simulink model "compressionGainBlock"  (R2019a)
settings: Solver=VariableStepAuto  StartTime=0.0  StopTime=t_end  RelTol=1e-3
InitFcn:
  | clear;
  | [sig, fs] = audioread('UnitStepVolumeTest.wav');
  | [Gain_Table, xp_spacing, max_gain] = ...
  |    Compression_Wrapper(fs, 0, 1, [1], [10], 85, 1);
  | Ts = 1/fs;
  | tt = (0:length(sig)-1)./fs;
  | t_end = tt(end);
  | sig_in = [tt', sig.*max_gain];
  | 
  | Table_Fill = zeros(1,length(tt))';
  | Table_Fill(1:64) = Gain_Table;
  | Table_Fill = [tt', Table_Fill];
  | Fill_Valid = zeros(1,length(tt))';
  | Fill_Valid(1:64) = ones(1,64)';
  | Fill_Valid = boolean(Fill_Valid);
  | Fill_Valid = [tt', Fill_Valid];
  | 
  | Reset = [tt', boolean(zeros(1,length(tt)))'];
  | 
  | t_att = 0.2; s_att = t_att*fs;
  | t_rel = 2.0; s_rel = t_rel*fs;
  | r_att = nthroot(0.1, s_att);
  | r_rel = nthroot(0.1, s_rel);
values from neighbouring files (symbols this model uses):
  sig = sig * 10.^(.05*adjustdB)    [loadwavfile.m]    (also in testing.m = X_sweep(Volume,:)')
  xp_spacing = (X_high-X_thresh)*max_gain_prescript/63    [Compression_Wrapper.m]
libraries: hdlsllib x2, simulink x1
settings Model: Creator=Bailey  LastModifiedBy=Bailey

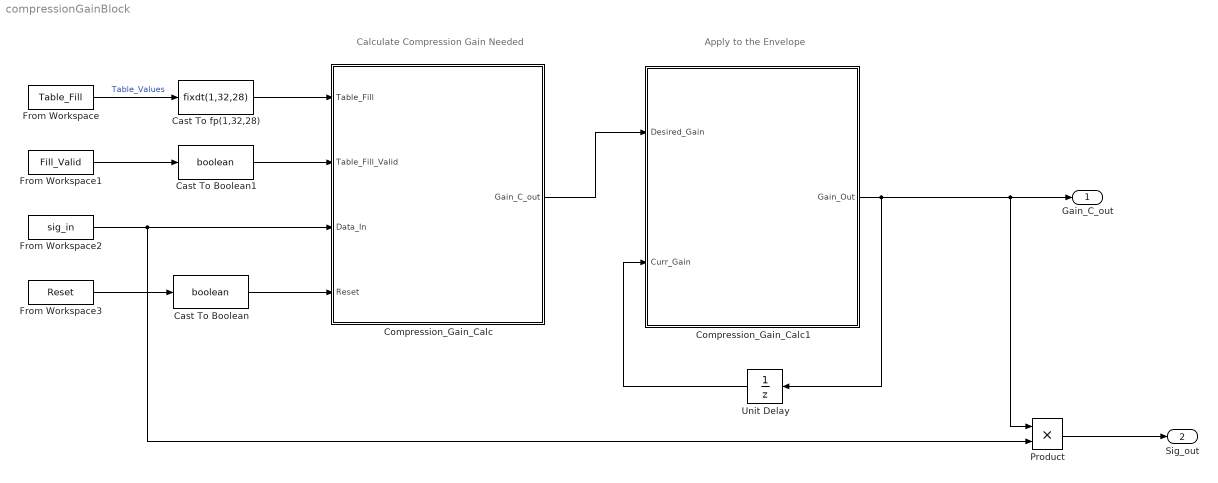
== system compressionGainBlock ==
  note: Apply to the Envelope
  note: Calculate Compression Gain Needed
  Cast To Boolean : DataTypeConversion  OutDataTypeStr=boolean
  Cast To Boolean1 : DataTypeConversion  OutDataTypeStr=boolean
  Cast To fp(1,32,28) : DataTypeConversion  OutDataTypeStr=fixdt(1,32,28)
  Compression_Gain_Calc : Subsystem
  Compression_Gain_Calc1 : Subsystem
  From Workspace : FromWorkspace  VariableName=Table_Fill  SampleTime=Ts  Interpolate=off  OutputAfterFinalValue=Setting to zero
  From Workspace1 : FromWorkspace  VariableName=Fill_Valid  SampleTime=Ts  OutputAfterFinalValue=Setting to zero
  From Workspace2 : FromWorkspace  VariableName=sig_in  SampleTime=Ts  Interpolate=off  OutputAfterFinalValue=Setting to zero
  From Workspace3 : FromWorkspace  VariableName=Reset  SampleTime=Ts  Interpolate=off  OutputAfterFinalValue=Setting to zero
  Product : Product
  Unit Delay : UnitDelay  InitialCondition=1  SampleTime=-1  HasFrameUpgradeWarning=on
  Gain_C_out : Outport
  Sig_out : Outport  Port=2
  wires:
  From Workspace2/1 -> Product/2, Compression_Gain_Calc/3(Data_In)
  From Workspace3/1 -> Cast To Boolean/1
  Cast To Boolean/1 -> Compression_Gain_Calc/4(Reset)
  From Workspace1/1 -> Cast To Boolean1/1
  Cast To Boolean1/1 -> Compression_Gain_Calc/2(Table_Fill_Valid)
  Cast To fp(1,32,28)/1 -> Compression_Gain_Calc/1(Table_Fill)
  From Workspace/1 -> Cast To fp(1,32,28)/1  "Table_Values"
  Compression_Gain_Calc/1(Gain_C_out) -> Compression_Gain_Calc1/1(Desired_Gain)
  Compression_Gain_Calc1/1(Gain_Out) -> Product/1, Gain_C_out/1, Unit Delay/1
  Unit Delay/1 -> Compression_Gain_Calc1/2(Curr_Gain)
  Product/1 -> Sig_out/1

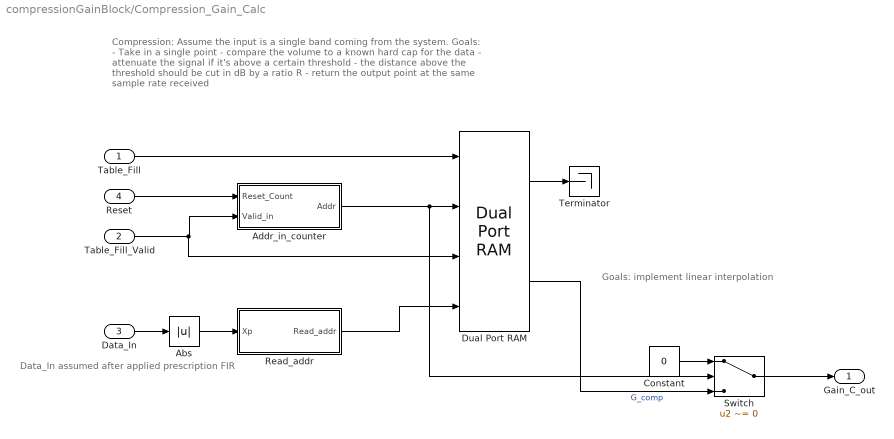
== system compressionGainBlock/Compression_Gain_Calc ==
  note: Goals: implement linear interpolation
  note: Data_In assumed after applied prescription FIR
  note: Compression: Assume the input is a single band coming from the system.
      |
      | Goals:
      | 	- Take in a single point
      | 	- compare the volume to a known hard cap for the data
      | 	- attenuate the signal if it's above a certain threshold
      | 		- the distance above the threshold should be cut in dB by a ratio R
      | 	- return the output point at the same sample rate received
  Table_Fill : Inport
  Table_Fill_Valid : Inport  Port=2
  Data_In : Inport  Port=3
  Reset : Inport  Port=4
  Abs : Abs
  Addr_in_counter : Subsystem
  Constant : Constant  Value=0  SampleTime=-1
  Dual Port RAM : hdlsllib/HDL RAMs/Dual Port RAM  ram_size=6
      settings: SourceProductName=Simulink  SourceProductBaseCode=SL
  Read_addr : Subsystem
  Switch : Switch  Criteria=u2 ~= 0  Threshold=63  ZeroCross=off
  Terminator : Terminator
  Gain_C_out : Outport
  wires:
  Reset/1 -> Addr_in_counter/1(Reset_Count)
  Dual Port RAM/1 -> Terminator/1
  Constant/1 -> Switch/1
  Switch/1 -> Gain_C_out/1
  Table_Fill/1 -> Dual Port RAM/1
  Table_Fill_Valid/1 -> Dual Port RAM/3, Addr_in_counter/2(Valid_in)
  Addr_in_counter/1(Addr) -> Switch/2, Dual Port RAM/2
  Dual Port RAM/2 -> Switch/3  "G_comp"
  Read_addr/1(Read_addr) -> Dual Port RAM/4
  Abs/1 -> Read_addr/1(Xp)
  Data_In/1 -> Abs/1

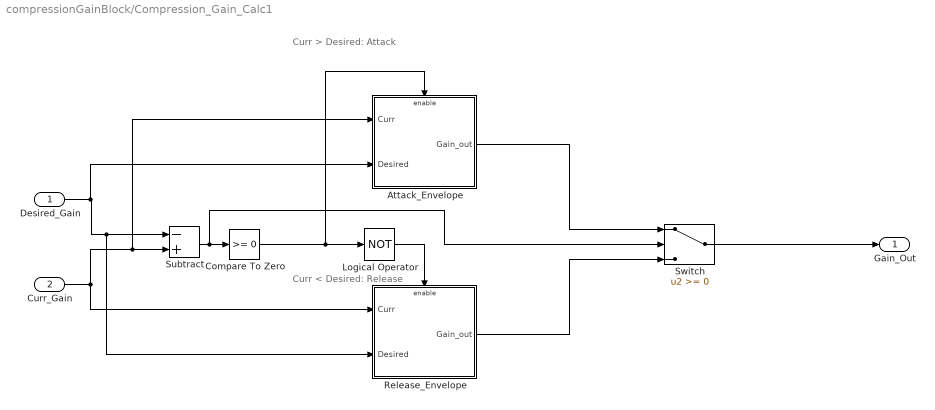
== system compressionGainBlock/Compression_Gain_Calc1 ==
  note: Curr > Desired:
      | Attack
  note: Curr < Desired:
      | Release
  Desired_Gain : Inport
  Curr_Gain : Inport  Port=2
  Attack_Envelope : Subsystem  TreatAsAtomicUnit=on
  Compare To Zero : simulink/Logic and Bit Operations/Compare To Zero  relop=>=  OutDataTypeStr=boolean
  Logical Operator : Logic  Operator=NOT  AllPortsSameDT=off  OutDataTypeStr=boolean
  Release_Envelope : Subsystem  TreatAsAtomicUnit=on
  Subtract : Sum  Inputs=-+
  Switch : Switch
  Gain_Out : Outport
  wires:
  Desired_Gain/1 -> Attack_Envelope/2(Desired), Release_Envelope/2(Desired), Subtract/1
  Curr_Gain/1 -> Attack_Envelope/1(Curr), Subtract/2, Release_Envelope/1(Curr)
  Subtract/1 -> Switch/2, Compare To Zero/1
  Compare To Zero/1 -> Attack_Envelope/Enable, Logical Operator/1
  Logical Operator/1 -> Release_Envelope/Enable
  Switch/1 -> Gain_Out/1
  Attack_Envelope/1(Gain_out) -> Switch/1
  Release_Envelope/1(Gain_out) -> Switch/3

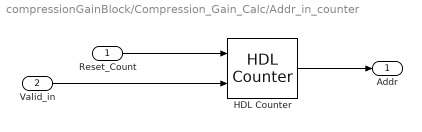
== system compressionGainBlock/Compression_Gain_Calc/Addr_in_counter ==
  Reset_Count : Inport
  Valid_in : Inport  Port=2
  HDL Counter : hdlsllib/Sources/HDL Counter  CountType=Count limited  CountInit=0  CountStep=1  CountMax=63  CountFromType=Initial value  CountFrom=0  CountResetPort=on  CountLoadPort=off  CountEnbPort=on  CountDirPort=off  CountDataType=Unsigned  CountWordLen=6  CountFracLen=0  CountSampTime=1
      settings: SourceProductName=Simulink
  Addr : Outport
  wires:
  Valid_in/1 -> HDL Counter/2
  Reset_Count/1 -> HDL Counter/1
  HDL Counter/1 -> Addr/1

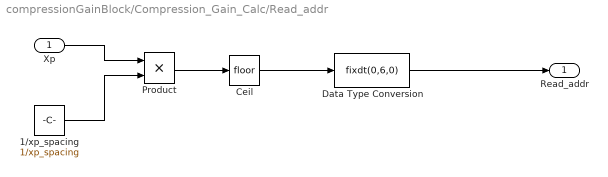
== system compressionGainBlock/Compression_Gain_Calc/Read_addr ==
  Xp : Inport
  1/xp_spacing : Constant  Value=1/xp_spacing  SampleTime=-1
  Ceil : Rounding
  Data Type Conversion : DataTypeConversion  OutDataTypeStr=fixdt(0,6,0)  RndMeth=Nearest
  Product : Product
  Read_addr : Outport
  wires:
  Xp/1 -> Product/1
  1/xp_spacing/1 -> Product/2
  Product/1 -> Ceil/1
  Ceil/1 -> Data Type Conversion/1
  Data Type Conversion/1 -> Read_addr/1

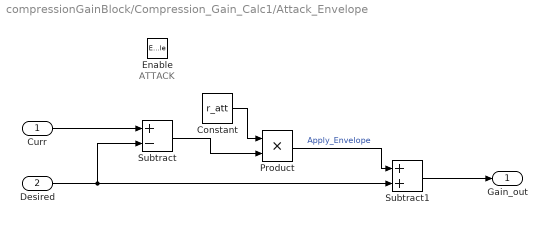
== system compressionGainBlock/Compression_Gain_Calc1/Attack_Envelope ==
  note: ATTACK
  Curr : Inport
  Desired : Inport  Port=2
  Enable : EnablePort
  Constant : Constant  Value=r_att  SampleTime=-1
  Product : Product
  Subtract : Sum  Inputs=+-
  Subtract1 : Sum
  Gain_out : Outport  InitialOutput=0
  wires:
  Desired/1 -> Subtract/2, Subtract1/2
  Curr/1 -> Subtract/1
  Subtract/1 -> Product/2
  Constant/1 -> Product/1
  Product/1 -> Subtract1/1  "Apply_Envelope"
  Subtract1/1 -> Gain_out/1

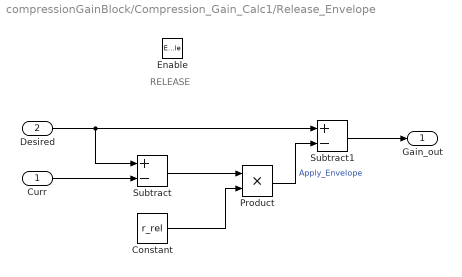
== system compressionGainBlock/Compression_Gain_Calc1/Release_Envelope ==
  note: RELEASE
  Curr : Inport
  Desired : Inport  Port=2
  Enable : EnablePort
  Constant : Constant  Value=r_rel  SampleTime=-1
  Product : Product
  Subtract : Sum  Inputs=+-
  Subtract1 : Sum  Inputs=+-
  Gain_out : Outport  InitialOutput=0
  wires:
  Desired/1 -> Subtract1/1, Subtract/1
  Curr/1 -> Subtract/2
  Subtract/1 -> Product/1
  Constant/1 -> Product/2
  Product/1 -> Subtract1/2  "Apply_Envelope"
  Subtract1/1 -> Gain_out/1
